simulink model "main"  (R2023a)
settings: Solver=ode45  StartTime=0.0  StopTime=100  FixedStep=0.05  RelTol=1e-3
values from neighbouring files (symbols this model uses):
  K_av = Ki_vel./Kp_vel    [regulator.m]
  Kd_pose = [Kd_pose_x, Kd_pose_y, Kd_pose_yaw]'    [regulator.m]
  Ki_vel = alpha * w_n^2    [regulator.m]
  Kp_pose = wn1* (Kd_pose+1)    [regulator.m]
  Kp_vel = Kp_vel    [regulator.m]
  wn1 = w_n /4    [regulator.m]
  x = 0    [regulator.m]
  y = 0    [regulator.m]
  yaw = pi/2    (= 1.57079632679)    [regulator.m]
libraries: MarineRoboticsLib x3
settings Model: Creator=thor  LastModifiedBy=Pero
settings OptimizationCC: ReuseModelBlockBuffer=off
settings DebuggingCC: UnconnectedInputMsg=warning  UnconnectedOutputMsg=warning  UnconnectedLineMsg=warning
settings ModelReferenceCC: EnableRefExpFcnMdlSchedulingChecks=on
settings RTWCC: DLArmComputeVersion=19.05

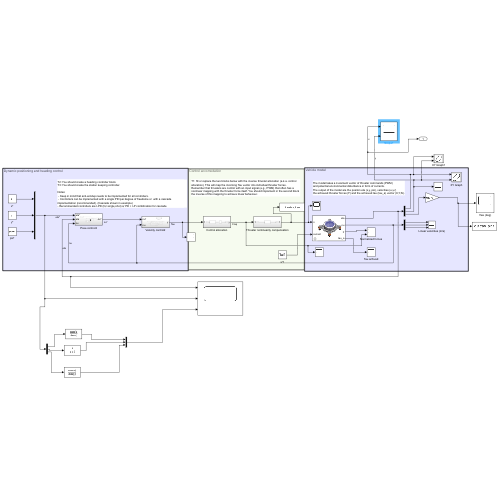
[thumbnail: Simulink's stored preview of the top-level diagram]
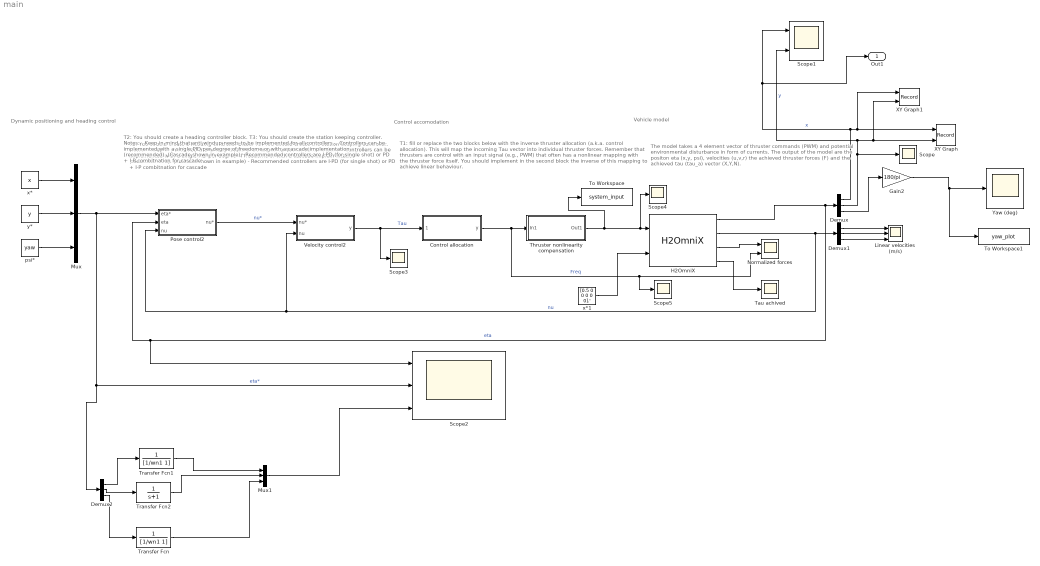
== system main ==
  note: T2: You should create a heading controller block.
      | T3: You should create the station keeping controller.
      |
      | Notes:
      |  - Keep in mind that anti-windup needs to be implemented for all controllers.
      |  - Controllers can be implemented with a single PID per degree of freedome or  with a cascade implementation (recommended). (Cascade shown in example)
      | - Recommended controllers are I-PD (for single shot) or PD + I-P combitnation for cascade
  note: Dynamic positioning and heading control
  note: T1: fill or replace the two blocks below with the inverse thruster allocation (a.k.a. control allocation). This will map the incoming Tau vector into individual thruster forces. Remember that thrusters are control with an input signal (e.g., PWM) that often has a nonlinear mapping with the thruster force itself. You should implement in the second block the inverse of this mapping to achieve linear behaviour.
  note: Vehicle model
  note: Control accomodation
  note: The model takes a 4 element vector of thruster commands (PWM)
      | and potential environmental disturbance in form of currents.
      | The output of the model are the positon eta (x,y, psi), velocities (u,v,r)
      | the achieved thruster forces (F) and the achieved tau (tau_a) vector (X,Y,N).
  note: T2: You should create a heading controller block.
      | T3: You should create the station keeping controller.
      |
      | Notes:
      |  - Keep in mind that anti-windup needs to be implemented for all controllers.
      |  - Controllers can be implemented with a single PID per degree of freedome or  with a cascade implementation (recommended). (Cascade shown in example)
      | - Recommended controllers are I-PD (for single shot) or PD + I-P combitnation for cascade
  Control allocation : Subsystem
  Demux : Demux  Outputs=3
  Demux1 : Demux  Outputs=3
  Demux2 : Demux  Outputs=3
  Gain2 : Gain  Gain=180/pi
  H2OmniX : MarineRoboticsLib/H2OmniX  alpha=[2.1,2.1,0.4]  beta=[1,1,0.24]  betaa=[0,0,0]  nu0=[0,0,0]  eta0=[0,0,0]
  Linear velocities (m/s) : Scope  NumInputPorts=3
  Mux : Mux  Inputs=3
  Mux1 : Mux  Inputs=3
  Normalized forces : Scope  NumInputPorts=2
  Pose control2 : Subsystem
  Scope{,3..5} (4 alike) : Scope
  Scope1 : Scope  NumInputPorts=2
  Scope2 : Scope  NumInputPorts=3
  Tau achived : Scope
  Thruster nonlinearity compensation : Subsystem
  To Workspace : ToWorkspace  VariableName=system_input  SaveFormat=Timeseries  SampleTime=-1
  To Workspace1 : ToWorkspace  VariableName=yaw_plot  SaveFormat=Timeseries  SampleTime=-1
  Transfer Fcn : TransferFcn  Numerator=[ 1]  Denominator=[1/wn1 1]
  Transfer Fcn1 : TransferFcn  Denominator=[1/wn1 1]
  Transfer Fcn2 : TransferFcn  Denominator=[1 1]
  Velocity control2 : Subsystem
  XY Graph : Record  FileSettingsInternal="{\"entries\":[{\"content\":{\"excelSettings\":{\"content\":{},\"type\":\"Streamout.ExcelSettings\"}},\"type\":\"Streamout.FileSettingStorage\",\"uuid\":\"\"}],\"packageUris\":[\"http:\\/\\/schema.mathworks.com\\/mf0\\/streamout_blocks\\/R2020a\"],\"version\":\"1.0\"}"  Layout=[1 1]  SignalsInternal="{\"entries\":[{\"content\":{\"signals\":[{\"content\":{\"blockPath\":[],\"dimensions\":[1],\"domain\":\"\",\"lineColor\":\"#a2142f\",\"plots\":[1],\"port\":1,\"sid\":[\"\"],\"signalID\":16314,\"signalName\":\"x\"},\"type\":\"RecordBlkView.Signal\",\"uuid\":\"\"},{\"content\":{\"blockPath\":[],\"dimensions\":[1],\"domain\":\"\",\"lineColor\":\"#139fff\",\"port\":2,\"sid\":[\"\"],\"signalID\":16318,\"signalName\":\"y\"},\"type\":\"RecordBlkView.Signal\",\"uuid\":\"\"}]},\"type\":\"RecordBlkView.InputSignals\",\"uuid\":\"\"}],\"packageUris\":[\"http:\\/\\/schema.mathworks.com\\/mf0\\/streamout_blocks\\/R2020a\"],\"version\":\"1.0\"}"  CompatibilityTag=XY
  XY Graph1 : Record  FileSettingsInternal="{\"entries\":[{\"content\":{\"excelSettings\":{\"content\":{},\"type\":\"Streamout.ExcelSettings\"}},\"type\":\"Streamout.FileSettingStorage\",\"uuid\":\"\"}],\"packageUris\":[\"http:\\/\\/schema.mathworks.com\\/mf0\\/streamout_blocks\\/R2020a\"],\"version\":\"1.0\"}"  Layout=[1 1]  SignalsInternal="{\"entries\":[{\"content\":{\"signals\":[{\"content\":{\"blockPath\":[],\"dimensions\":[1],\"domain\":\"\",\"lineColor\":\"#a2142f\",\"plots\":[1],\"port\":1,\"sid\":[\"\"],\"signalID\":16322,\"signalName\":\"x\"},\"type\":\"RecordBlkView.Signal\",\"uuid\":\"\"},{\"content\":{\"blockPath\":[],\"dimensions\":[1],\"domain\":\"\",\"lineColor\":\"#139fff\",\"plots\":[1],\"port\":2,\"sid\":[\"\"],\"signalID\":16326,\"signalName\":\"y\"},\"type\":\"RecordBlkView.Signal\",\"uuid\":\"\"}]},\"type\":\"RecordBlkView.InputSignals\",\"uuid\":\"\"}],\"packageUris\":[\"http:\\/\\/schema.mathworks.com\\/mf0\\/streamout_blocks\\/R2020a\"],\"version\":\"1.0\"}"  VisualizationBindings="{\"xyplotplugin\":{\"info\":[{\"series\":[{\"bindingParametersList\":[{\"parameter\":\"X-Axis\",\"signalID\":16322,\"signalName\":\"x\"},{\"parameter\":\"Y-Axis\",\"signalID\":16326,\"signalName\":\"y\"}],\"seriesID\":11065}],\"subplotID\":1}]}}"  CompatibilityTag=XY
  Yaw (deg) : Scope
  psi* : Constant  Value=yaw
  x* : Constant  Value=x
  x*1 : Constant  Value=[0.5 0 0 0 0 0].'
  y* : Constant  Value=y
  Out1 : Outport
  wires:
  H2OmniX/1 -> Demux/1, Pose control2/2(eta), Scope2/1  "eta"
  Demux/1 -> XY Graph1/1, XY Graph/1, Out1/1, Scope1/1  "x"
  Demux/2 -> Scope/1, XY Graph1/2, XY Graph/2, Scope1/2  "y"
  H2OmniX/2 -> Velocity control2/2(nu), Pose control2/3(nu), Demux1/1  "nu"
  Demux1/1 -> Linear velocities (m/s)/1
  Demux1/2 -> Linear velocities (m/s)/2
  Demux1/3 -> Linear velocities (m/s)/3
  Demux/3 -> Gain2/1
  Gain2/1 -> To Workspace1/1, Yaw (deg)/1
  H2OmniX/3 -> Normalized forces/1
  H2OmniX/4 -> Tau achived/1
  Control allocation/1(y) -> Scope5/1, Normalized forces/2, Thruster nonlinearity compensation/1(In1)  "Freq"
  Thruster nonlinearity compensation/1(Out1) -> To Workspace/1, Scope4/1, H2OmniX/1
  Velocity control2/1(y) -> Scope3/1, Control allocation/1(1)  "Tau"
  Pose control2/1(nu*) -> Velocity control2/1(nu*)  "nu*"
  Mux/1 -> Pose control2/1(eta*), Demux2/1, Scope2/2  "eta*"
  x*/1 -> Mux/1
  y*/1 -> Mux/2
  psi*/1 -> Mux/3
  Demux2/1 -> Transfer Fcn1/1
  Demux2/2 -> Transfer Fcn2/1
  Demux2/3 -> Transfer Fcn/1
  Transfer Fcn/1 -> Mux1/3
  Transfer Fcn1/1 -> Mux1/1
  Transfer Fcn2/1 -> Mux1/2
  Mux1/1 -> Scope2/3
  x*1/1 -> H2OmniX/2

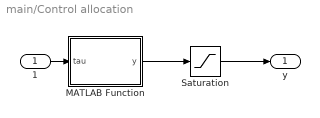
== system main/Control allocation ==
  1 : Inport
  MATLAB Function : MATLAB Function  TreatAsAtomicUnit=on
  Saturation : Saturate  UpperLimit=0.85  LowerLimit=-0.85
  y : Outport
  wires:
  1/1 -> MATLAB Function/1(tau)
  MATLAB Function/1(y) -> Saturation/1
  Saturation/1 -> y/1

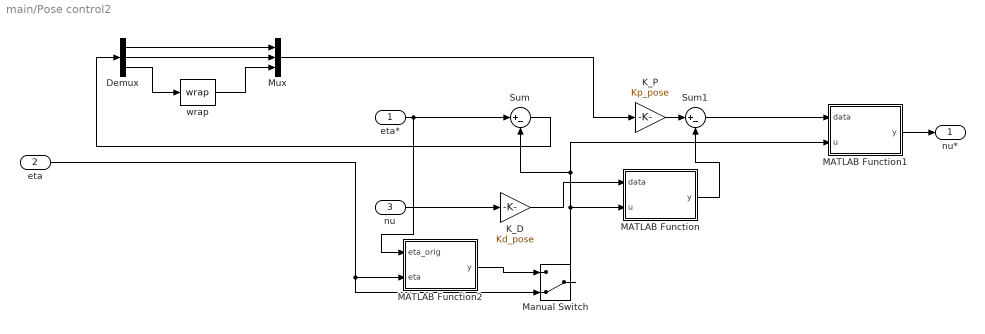
== system main/Pose control2 ==
  eta* : Inport
  eta : Inport  Port=2
  nu : Inport  Port=3
  Demux : Demux  Outputs=3
  K_D : Gain  Gain=Kd_pose
  K_P : Gain  Gain=Kp_pose
  MATLAB Function : MATLAB Function  TreatAsAtomicUnit=on
  MATLAB Function1 : MATLAB Function  TreatAsAtomicUnit=on
  MATLAB Function2 : MATLAB Function  TreatAsAtomicUnit=on
  Manual Switch : ManualSwitch  CurrentSetting=0
  Mux : Mux  Inputs=3
  Sum : Sum  Inputs=|+-
  Sum1 : Sum  Inputs=|+-
  wrap : MarineRoboticsLib/H2OmniX/wrap  SystemSampleTime=-1  VariantActivationTime=update diagram  Latency=0  AutoFrameSizeCalculation=off
      settings: LibrarySourceBlock=|
      | simulink/User-Defined
      | Functions/MATLAB Function
  nu* : Outport
  wires:
  eta*/1 -> MATLAB Function2/1(eta_orig), Sum/1
  nu/1 -> K_D/1
  K_D/1 -> MATLAB Function/1(data)
  MATLAB Function/1(y) -> Sum1/2
  MATLAB Function1/1(y) -> nu*/1
  eta/1 -> Manual Switch/2, MATLAB Function2/2(eta)
  MATLAB Function2/1(y) -> Manual Switch/1
  Manual Switch/1 -> MATLAB Function/2(u), MATLAB Function1/2(u), Sum/2
  Sum1/1 -> MATLAB Function1/1(data)
  K_P/1 -> Sum1/1
  Demux/1 -> Mux/1
  Demux/2 -> Mux/2
  Demux/3 -> wrap/1
  wrap/1 -> Mux/3
  Sum/1 -> Demux/1
  Mux/1 -> K_P/1

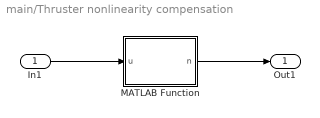
== system main/Thruster nonlinearity compensation ==
  In1 : Inport
  MATLAB Function : MATLAB Function  TreatAsAtomicUnit=on
  Out1 : Outport
  wires:
  In1/1 -> MATLAB Function/1(u)
  MATLAB Function/1(n) -> Out1/1

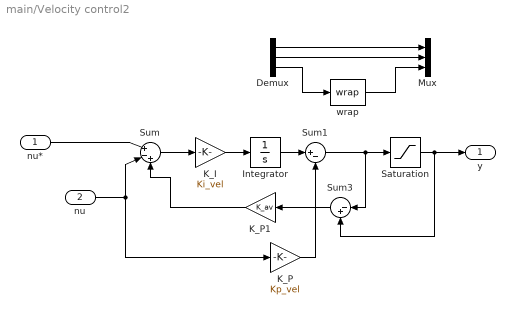
== system main/Velocity control2 ==
  nu* : Inport
  nu : Inport  Port=2
  Demux : Demux  Outputs=3
  Integrator : Integrator
  K_I : Gain  Gain=Ki_vel
  K_P : Gain  Gain=Kp_vel
  K_P1 : Gain  Gain=K_av
  Mux : Mux  Inputs=3
  Saturation : Saturate  UpperLimit=0.85  LowerLimit=-0.85
  Sum : Sum  Inputs=|+-+
  Sum1 : Sum  Inputs=|+-
  Sum3 : Sum  Inputs=|-+
  wrap : MarineRoboticsLib/H2OmniX/wrap  SystemSampleTime=-1  VariantActivationTime=update diagram  Latency=0  AutoFrameSizeCalculation=off
      settings: LibrarySourceBlock=|
      | simulink/User-Defined
      | Functions/MATLAB Function
  y : Outport
  wires:
  nu*/1 -> Sum/1
  nu/1 -> K_P/1, Sum/2
  K_P/1 -> Sum1/2
  Sum1/1 -> Sum3/1, Saturation/1
  Saturation/1 -> y/1, Sum3/2
  Integrator/1 -> Sum1/1
  Sum3/1 -> K_P1/1
  K_I/1 -> Integrator/1
  K_P1/1 -> Sum/3
  Demux/1 -> Mux/1
  Demux/3 -> wrap/1
  Demux/2 -> Mux/2
  wrap/1 -> Mux/3
  Sum/1 -> K_I/1

== matlab function main/Control allocation/MATLAB Function ==
  data: tau input; y output
function y = fcn(tau)

B = [0.25, 0.25, -0.25, -0.25; -0.25,  0.25, -0.25,  0.25; -0.25, 0.25, 0.25, -0.25];

y = pinv(B)*tau;

end

== matlab function main/Pose control2/MATLAB Function ==
  data: data input; u input; y output
function y = fcn(data, u)
%data = [u, v, d_psi]
%u = [x, y, psi]
psi = u(3);
R = [cos(psi), -sin(psi), 0;
     sin(psi), cos(psi),  0;
        0,         0,     1];
y = R*data;

== matlab function main/Pose control2/MATLAB Function1 ==
  data: data input; u input; y output
function y = fcn(data, u)
%data = [u, v, d_psi]
%u = [x, y, psi]
psi = u(3);
R = [cos(psi), -sin(psi), 0;
     sin(psi), cos(psi),  0;
        0,         0,     1];
y = R'*data;

== matlab function main/Pose control2/MATLAB Function2 ==
  data: eta_orig input; eta input size=3; y output
function y   = fcn(eta_orig , eta )

if abs(eta_orig(1) - eta(1)) < 0.2 | abs(eta_orig(2) - eta(2)) < 0.2 
    y = eta_orig;
else
    y = eta;
end
end

== matlab function main/Thruster nonlinearity compensation/MATLAB Function ==
  data: u input; n output
function n = fcn(u)

for i = 1:length(u)
    if u(i) > 1
        u(i) = 1;
    end
end

p1 = 0.5869;
p2 = -0.9109;
p3 = -0.3809;
p4 = 1.6743;
p5 = -0.0089;

n = p1*u.^4 + p2*u.^3 + p3*u.^2 + p4*u + p5;
